simulink library "ACT_MTR"  (Simulink 10.2)
settings: Solver=VariableStepAuto  StartTime=0.0  StopTime=10.0  RelTol=1e-3
settings Model: Creator=dbell44  LastModifiedBy=dbell44

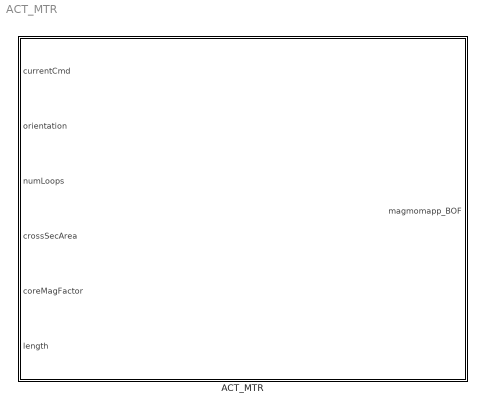
== system ACT_MTR ==
  ACT_MTR : Subsystem

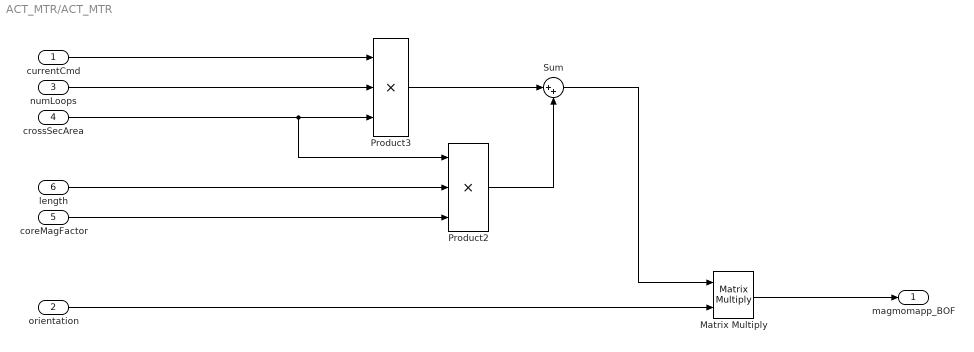
== system ACT_MTR/ACT_MTR ==
  currentCmd : Inport
  orientation : Inport  Port=2
  numLoops : Inport  Port=3
  crossSecArea : Inport  Port=4
  coreMagFactor : Inport  Port=5
  length : Inport  Port=6
  Matrix Multiply : Product  Multiplication=Matrix(*)
  Product2 : Product  Inputs=3
  Product3 : Product  Inputs=3
  Sum : Sum  Inputs=|++
  magmomapp_BOF : Outport
  wires:
  orientation/1 -> Matrix Multiply/2
  length/1 -> Product2/2
  currentCmd/1 -> Product3/1
  numLoops/1 -> Product3/2
  Matrix Multiply/1 -> magmomapp_BOF/1
  Product2/1 -> Sum/2
  Product3/1 -> Sum/1
  coreMagFactor/1 -> Product2/3
  Sum/1 -> Matrix Multiply/1
  crossSecArea/1 -> Product3/3, Product2/1
